simulink model "State_space_validation"  (R2024b)
settings: Solver=FixedStepAuto  StartTime=0.0  StopTime=40  FixedStep=0.0001  RelTol=1e-3
undefined symbols (not defined in the file): daq, degs2rpm, drv, gbox, K, Kff, mld, mot, rads2rpm, rdp, rpm2rads, sens, step_gain, Ts, u_bar_max
settings Model: Creator=Enrico  LastModifiedBy=farin
settings DataIOCC: ReturnWorkspaceOutputsName=out_black_box

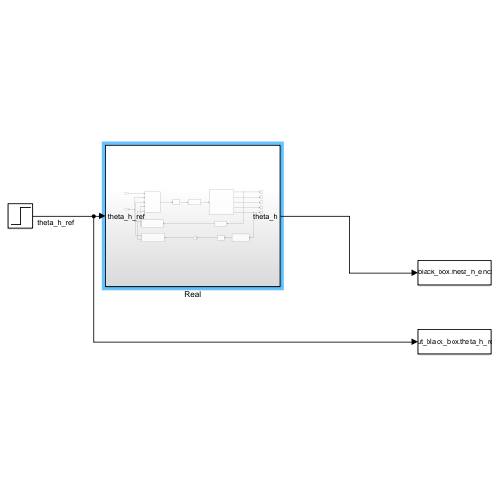
[thumbnail: Simulink's stored preview of the top-level diagram]
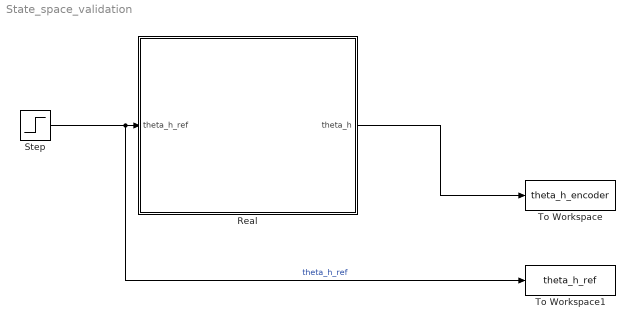
== system State_space_validation ==
  Real : Subsystem
  Step : Step  After=step_gain  SampleTime=0
  To Workspace : ToWorkspace  VariableName=theta_h_encoder  SaveFormat=Structure With Time  SampleTime=-1
  To Workspace1 : ToWorkspace  VariableName=theta_h_ref  SaveFormat=Structure With Time  SampleTime=-1
  wires:
  Step/1 -> To Workspace1/1, Real/1(theta_h_ref)  "theta_h_ref"
  Real/1(theta_h) -> To Workspace/1

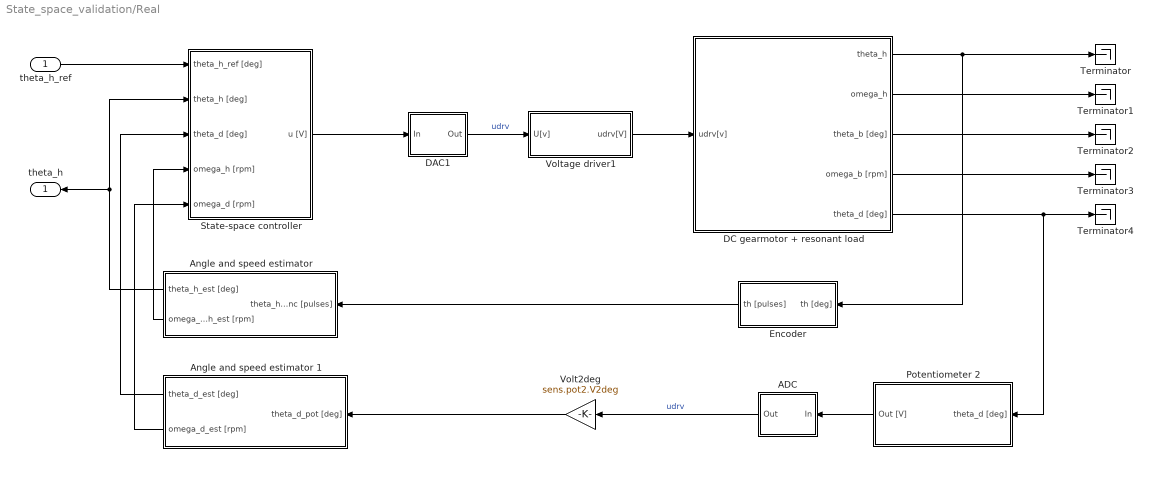
== system State_space_validation/Real ==
  theta_h_ref : Inport
  ADC : Subsystem
  Angle and speed estimator : Subsystem
  Angle and speed estimator 1 : Subsystem
  DAC1 : Subsystem
  DC gearmotor + resonant load : Subsystem
  Encoder : Subsystem
  Potentiometer 2 : Subsystem
  State-space controller : Subsystem
  Terminator{,1..4} (5 alike) : Terminator
  Volt2deg : Gain  Gain=sens.pot2.V2deg
  Voltage driver1 : Subsystem
  theta_h : Outport
  wires:
  DC gearmotor + resonant load/1(theta_h) -> Terminator/1, Encoder/1(th [deg])
  DC gearmotor + resonant load/5(theta_d [deg]) -> Potentiometer 2/1(theta_d [deg]), Terminator4/1
  DC gearmotor + resonant load/4(omega_b [rpm]) -> Terminator3/1
  Voltage driver1/1(udrv[V]) -> DC gearmotor + resonant load/1(udrv[v])
  DAC1/1(Out) -> Voltage driver1/1(U[v])  "udrv"
  DC gearmotor + resonant load/2(omega_h) -> Terminator1/1
  DC gearmotor + resonant load/3(theta_b [deg]) -> Terminator2/1
  Potentiometer 2/1(Out [V]) -> ADC/1(In)
  ADC/1(Out) -> Volt2deg/1  "udrv"
  State-space controller/1(u [V]) -> DAC1/1(In)
  Volt2deg/1 -> Angle and speed estimator 1/1(theta_d_pot [deg])
  Encoder/1(th [pulses]) -> Angle and speed estimator/1(theta_h_enc [pulses])
  Angle and speed estimator/1(theta_h_est [deg]) -> State-space controller/2(theta_h [deg]), theta_h/1
  Angle and speed estimator/2(omega_h_est [rpm]) -> State-space controller/4(omega_h [rpm])
  Angle and speed estimator 1/1(theta_d_est [deg]) -> State-space controller/3(theta_d [deg])
  Angle and speed estimator 1/2(omega_d_est [rpm]) -> State-space controller/5(omega_d [rpm])
  theta_h_ref/1 -> State-space controller/1(theta_h_ref [deg])

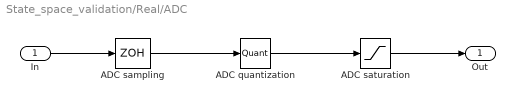
== system State_space_validation/Real/ADC ==
  In : Inport
  ADC quantization : Quantizer  QuantizationInterval=daq.adc.q
  ADC sampling : ZeroOrderHold  SampleTime=Ts
  ADC saturation : Saturate  UpperLimit=daq.adc.fs  LowerLimit=-daq.adc.fs
  Out : Outport
  wires:
  ADC quantization/1 -> ADC saturation/1
  In/1 -> ADC sampling/1
  ADC sampling/1 -> ADC quantization/1
  ADC saturation/1 -> Out/1

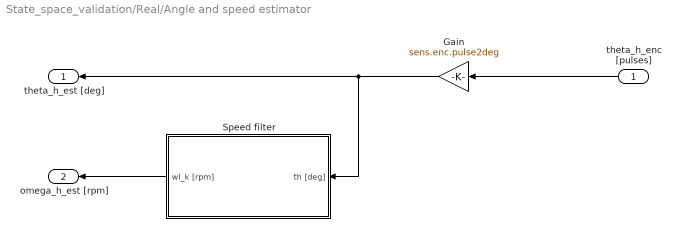
== system State_space_validation/Real/Angle and speed estimator ==
  theta_h_enc [pulses] : Inport
  Gain : Gain  Gain=sens.enc.pulse2deg
  Speed filter : Subsystem
  theta_h_est [deg] : Outport
  omega_h_est [rpm] : Outport  Port=2
  wires:
  Speed filter/1(wl_k [rpm]) -> omega_h_est [rpm]/1
  theta_h_enc [pulses]/1 -> Gain/1
  Gain/1 -> Speed filter/1(th [deg]), theta_h_est [deg]/1

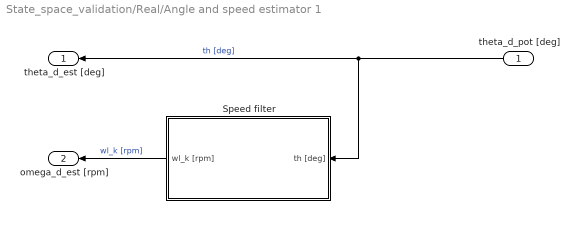
== system State_space_validation/Real/Angle and speed estimator 1 ==
  theta_d_pot [deg] : Inport
  Speed filter : Subsystem
  theta_d_est [deg] : Outport
  omega_d_est [rpm] : Outport  Port=2
  wires:
  Speed filter/1(wl_k [rpm]) -> omega_d_est [rpm]/1  "wl_k [rpm]"
  theta_d_pot [deg]/1 -> Speed filter/1(th [deg]), theta_d_est [deg]/1  "th [deg]"

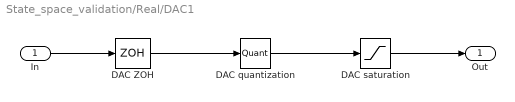
== system State_space_validation/Real/DAC1 ==
  In : Inport
  DAC ZOH : ZeroOrderHold  SampleTime=Ts
  DAC quantization : Quantizer  QuantizationInterval=daq.dac.q
  DAC saturation : Saturate  UpperLimit=daq.dac.fs  LowerLimit=-daq.dac.fs
  Out : Outport
  wires:
  DAC quantization/1 -> DAC saturation/1
  In/1 -> DAC ZOH/1
  DAC ZOH/1 -> DAC quantization/1
  DAC saturation/1 -> Out/1

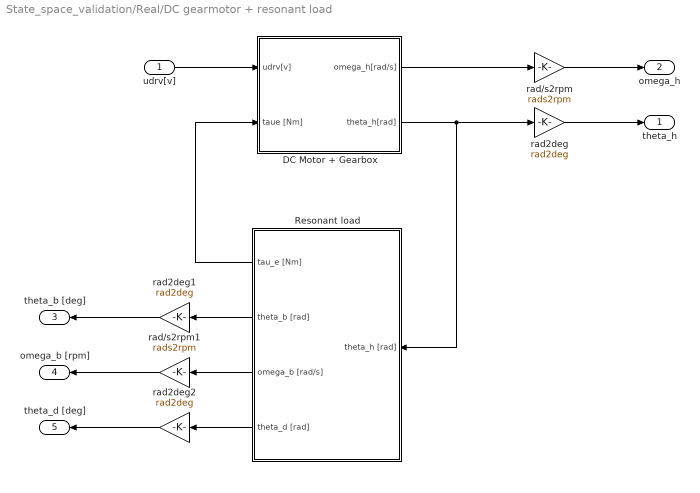
== system State_space_validation/Real/DC gearmotor + resonant load ==
  udrv[v] : Inport
  DC Motor + Gearbox : Subsystem
  Resonant load : Subsystem
  rad/s2rpm : Gain  Gain=rads2rpm
  rad/s2rpm1 : Gain  Gain=rads2rpm
  rad2deg : Gain  Gain=rad2deg
  rad2deg1 : Gain  Gain=rad2deg
  rad2deg2 : Gain  Gain=rad2deg
  theta_h : Outport
  omega_h : Outport  Port=2
  theta_b [deg] : Outport  Port=3
  omega_b [rpm] : Outport  Port=4
  theta_d [deg] : Outport  Port=5
  wires:
  udrv[v]/1 -> DC Motor + Gearbox/1(udrv[v])
  DC Motor + Gearbox/2(theta_h[rad]) -> rad2deg/1, Resonant load/1(theta_h [rad])
  Resonant load/3(omega_b [rad/s]) -> rad/s2rpm1/1
  Resonant load/2(theta_b [rad]) -> rad2deg1/1
  Resonant load/1(tau_e [Nm]) -> DC Motor + Gearbox/2(taue [Nm])
  rad/s2rpm1/1 -> omega_b [rpm]/1
  rad2deg2/1 -> theta_d [deg]/1
  rad2deg1/1 -> theta_b [deg]/1
  Resonant load/4(theta_d [rad]) -> rad2deg2/1
  rad/s2rpm/1 -> omega_h/1
  DC Motor + Gearbox/1(omega_h[rad/s]) -> rad/s2rpm/1
  rad2deg/1 -> theta_h/1

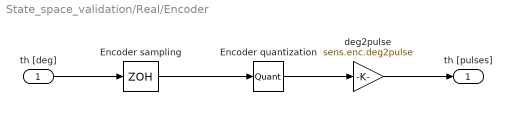
== system State_space_validation/Real/Encoder ==
  th [deg] : Inport
  Encoder quantization : Quantizer  QuantizationInterval=sens.enc.pulse2deg
  Encoder sampling : ZeroOrderHold  SampleTime=Ts
  deg2pulse : Gain  Gain=sens.enc.deg2pulse
  th [pulses] : Outport
  wires:
  Encoder quantization/1 -> deg2pulse/1
  th [deg]/1 -> Encoder sampling/1
  Encoder sampling/1 -> Encoder quantization/1
  deg2pulse/1 -> th [pulses]/1

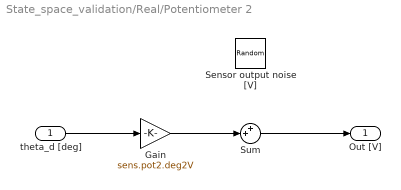
== system State_space_validation/Real/Potentiometer 2 ==
  theta_d [deg] : Inport
  Gain : Gain  Gain=sens.pot2.deg2V
  Sensor output noise [V] : RandomNumber  SampleTime=Ts
  Sum : Sum  Inputs=++|
  Out [V] : Outport
  wires:
  theta_d [deg]/1 -> Gain/1
  Sum/1 -> Out [V]/1
  Gain/1 -> Sum/2

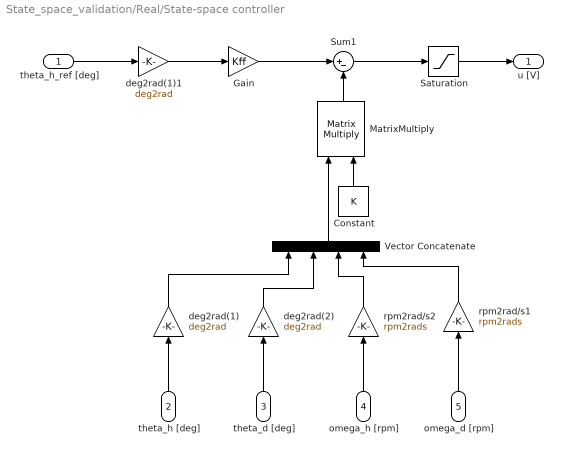
== system State_space_validation/Real/State-space controller ==
  theta_h_ref [deg] : Inport
  theta_h [deg] : Inport  Port=2
  theta_d [deg] : Inport  Port=3
  omega_h [rpm] : Inport  Port=4
  omega_d [rpm] : Inport  Port=5
  Constant : Constant  Value=K
  Gain : Gain  Gain=Kff
  MatrixMultiply : Product  Multiplication=Matrix(*)
  Saturation : Saturate  UpperLimit=u_bar_max  LowerLimit=-u_bar_max
  Sum1 : Sum  Inputs=|+-
  Vector Concatenate : Concatenate  NumInputs=4
  deg2rad(1) : Gain  Gain=deg2rad
  deg2rad(1)1 : Gain  Gain=deg2rad
  deg2rad(2) : Gain  Gain=deg2rad
  rpm2rad/s1 : Gain  Gain=rpm2rads
  rpm2rad/s2 : Gain  Gain=rpm2rads
  u [V] : Outport
  wires:
  deg2rad(2)/1 -> Vector Concatenate/2
  theta_h [deg]/1 -> deg2rad(1)/1
  Gain/1 -> Sum1/1
  deg2rad(1)/1 -> Vector Concatenate/1
  Constant/1 -> MatrixMultiply/2
  omega_d [rpm]/1 -> rpm2rad/s1/1
  rpm2rad/s2/1 -> Vector Concatenate/3
  rpm2rad/s1/1 -> Vector Concatenate/4
  Vector Concatenate/1 -> MatrixMultiply/1
  MatrixMultiply/1 -> Sum1/2
  theta_d [deg]/1 -> deg2rad(2)/1
  omega_h [rpm]/1 -> rpm2rad/s2/1
  deg2rad(1)1/1 -> Gain/1
  theta_h_ref [deg]/1 -> deg2rad(1)1/1
  Saturation/1 -> u [V]/1
  Sum1/1 -> Saturation/1

== system State_space_validation/Real/Voltage driver1 ==
  U[v] : Inport
  Driver dynamics : TransferFcn  Numerator=[drv.dcgain]  Denominator=[drv.Tc 1]
  Driver saturation : Saturate  UpperLimit=12  LowerLimit=-12
  udrv[V] : Outport
  wires:
  U[v]/1 -> Driver dynamics/1
  Driver dynamics/1 -> Driver saturation/1
  Driver saturation/1 -> udrv[V]/1

== system State_space_validation/Real/Angle and speed estimator/Speed filter ==
  th [deg] : Inport
  Real Derivative : TransferFcn  Numerator=[rdp.wci^2 0]  Denominator=[1 2*rdp.di*rdp.wci rdp.wci^2]
  degs2rpm : Gain  Gain=degs2rpm
  wl_k [rpm] : Outport
  wires:
  th [deg]/1 -> Real Derivative/1
  degs2rpm/1 -> wl_k [rpm]/1  "wl-meas"
  Real Derivative/1 -> degs2rpm/1

== system State_space_validation/Real/Angle and speed estimator 1/Speed filter ==
  th [deg] : Inport
  Real Derivative : TransferFcn  Numerator=[rdp.wci^2 0]  Denominator=[1 2*rdp.di*rdp.wci rdp.wci^2]
  degs2rpm : Gain  Gain=degs2rpm
  wl_k [rpm] : Outport
  wires:
  th [deg]/1 -> Real Derivative/1
  degs2rpm/1 -> wl_k [rpm]/1  "wl-meas"
  Real Derivative/1 -> degs2rpm/1

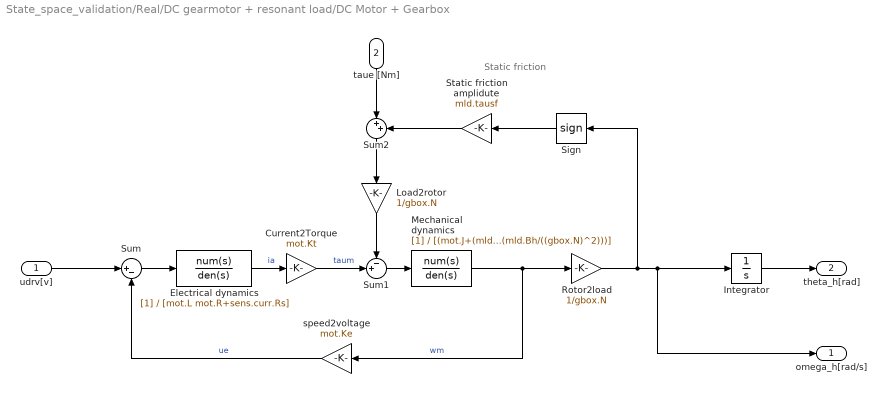
== system State_space_validation/Real/DC gearmotor + resonant load/DC Motor + Gearbox ==
  note: Static friction
  udrv[v] : Inport
  taue [Nm] : Inport  Port=2
  " Sign" : Signum  ZeroCross=off
  Current2Torque : Gain  Gain=mot.Kt
  Electrical dynamics : TransferFcn  Denominator=[mot.L mot.R+sens.curr.Rs]
  Integrator : Integrator
  Load2rotor : Gain  Gain=1/gbox.N
  Mechanical dynamics : TransferFcn  Denominator=[(mot.J+(mld.Jh/((gbox.N)^2))) (mot.B+(mld.Bh/((gbox.N)^2)))]
  Rotor2load : Gain  Gain=1/gbox.N
  Static friction amplidute : Gain  Gain=mld.tausf
  Sum : Sum  Inputs=|+-
  Sum1 : Sum  Inputs=-+|
  Sum2 : Sum  Inputs=|++
  speed2voltage : Gain  Gain=mot.Ke
  omega_h[rad/s] : Outport
  theta_h[rad] : Outport  Port=2
  wires:
  udrv[v]/1 -> Sum/1
  Sum/1 -> Electrical dynamics/1
  Electrical dynamics/1 -> Current2Torque/1  "ia"
  Current2Torque/1 -> Sum1/2  "taum"
  Load2rotor/1 -> Sum1/1
  " Sign"/1 -> Static friction amplidute/1
  Sum1/1 -> Mechanical dynamics/1
  Mechanical dynamics/1 -> speed2voltage/1, Rotor2load/1  "wm"
  speed2voltage/1 -> Sum/2  "ue"
  Rotor2load/1 -> " Sign"/1, omega_h[rad/s]/1, Integrator/1
  Sum2/1 -> Load2rotor/1
  Static friction amplidute/1 -> Sum2/2
  taue [Nm]/1 -> Sum2/1
  Integrator/1 -> theta_h[rad]/1

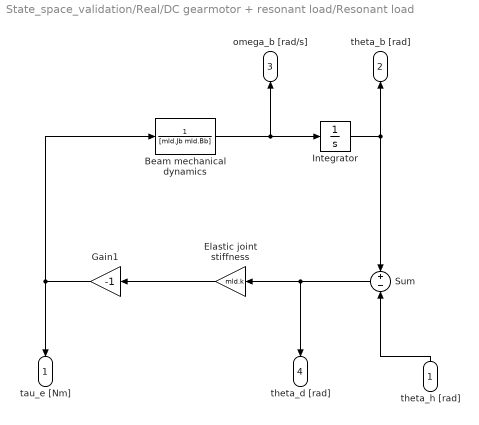
== system State_space_validation/Real/DC gearmotor + resonant load/Resonant load ==
  theta_h [rad] : Inport
  Beam mechanical dynamics : TransferFcn  Denominator=[mld.Jb mld.Bb]
  Elastic joint stiffness : Gain  Gain=mld.k
  Gain1 : Gain  Gain=-1
  Integrator : Integrator
  Sum : Sum  Inputs=+|-
  tau_e [Nm] : Outport
  theta_b [rad] : Outport  Port=2
  omega_b [rad/s] : Outport  Port=3
  theta_d [rad] : Outport  Port=4
  wires:
  theta_h [rad]/1 -> Sum/2
  Gain1/1 -> tau_e [Nm]/1, Beam mechanical dynamics/1
  Sum/1 -> Elastic joint stiffness/1, theta_d [rad]/1
  Integrator/1 -> theta_b [rad]/1, Sum/1
  Elastic joint stiffness/1 -> Gain1/1
  Beam mechanical dynamics/1 -> omega_b [rad/s]/1, Integrator/1
